simulink model "Hospital_Context"  (R2025b)
settings: Solver=VariableStepAuto  StartTime=0.0  StopTime=10.0  RelTol=1e-3
settings Model: Creator=jakeo  LastModifiedBy=jakeo

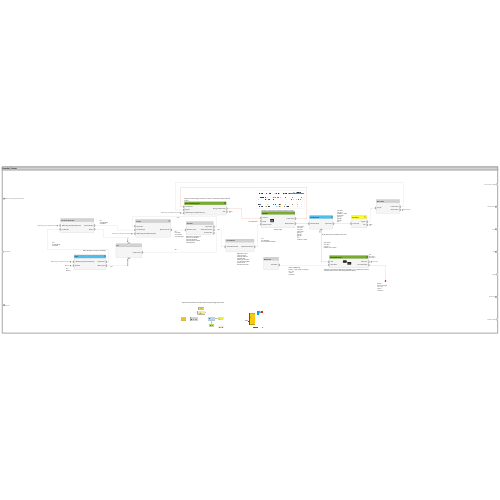
[thumbnail: Simulink's stored preview of the top-level diagram]
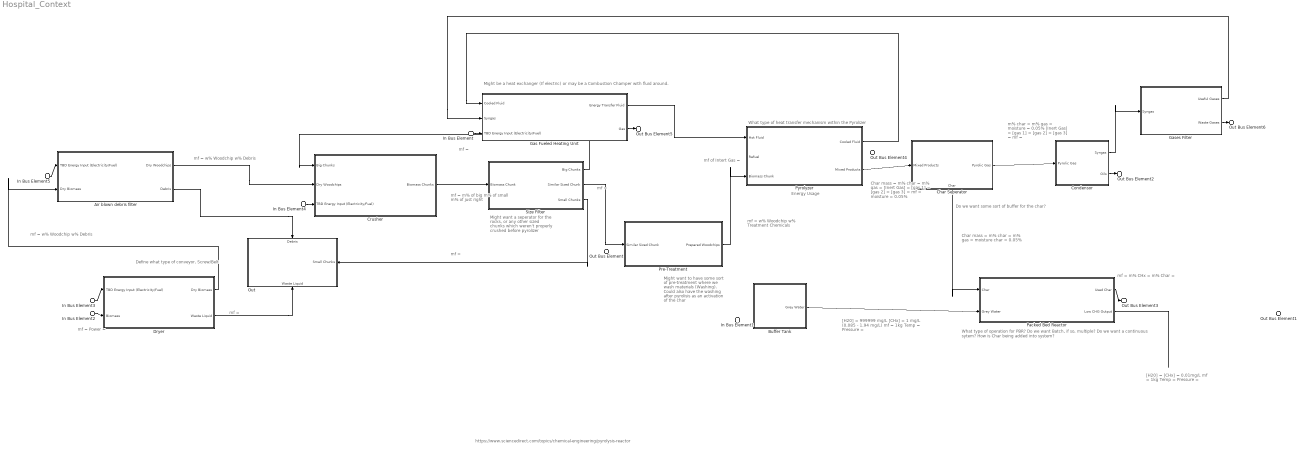
== system Hospital_Context ==
  note: mf =
      | m% CHx =
      | m% Char =
  note: Energy Usage
  note: mf of Intert Gas =
  note: m% char =
      | m% gas =
      | moisture = 0.05%
      | [Inert Gas] =
      | [gas 1] =
      | [gas 2] =
      | [gas 3] =
      | mf =
  note: Char mass =
      | m% char =
      | m% gas =
      | moisture char = 0.05%
  note: mf =
      | Power =
  note: Might want to have some sort of pre-treatment where we wash materials (Washing). Could also have the washing after pyrolisis as an activation of the char
  note: Do we want some sort of buffer for the char?
  note: What type of operation for PBR? Do we want Batch, if so, multiple? Do we want a continuous sytem? How is Char being added into system?
  note: Might want a seperator for the rocks, or any other sized chunks which weren't properly crushed before pyrolizer
  note: What type of heat transfer mechanism within the Pyrolizer
  note: Define what type of conveyor, Screw/Belt
  note: Might be a heat exchanger (If electric) or may be a Combustion Champer with fluid around.
  note: https://www.sciencedirect.com/topics/chemical-engineering/pyrolysis-reactor
  note: [H20] = 999999 mg/L
      | [CHx] = 1 mg/L  (0.085 - 1.94 mg/L)
      | mf = 1kg
      | Temp =
      | Pressure =
  note: [H20] =
      | [CHx] = 0.01mg/L
      | mf = 1kg
      | Temp =
      | Pressure =
  note: mf =
  note: mf =
      | w% Woodchip
      | w% Debris
  note: mf =
      | w% Woodchip
      | w% Debris
  note: Char mass =
      | m% char =
      | m% gas =
      | [Inert Gas] =
      | [gas 1] =
      | [gas 2] =
      | [gas 3] =
      | mf =
      | moisture = 0.05%
  note: mf =
      | m% of big
      | m% of small
      | m% of just right
  note: mf =
  note: mf =
      | w% Woodchip
      | w% Treatment Chemicals
  note: mf =
  note: mf =
  In Bus Element{,3..5} (4 alike) : Inport  PortName=TBD Energy Input (Electricity/Fuel)
  In Bus Element1 : Inport  Port=2  PortName=Grey Water 1
  In Bus Element2 : Inport  Port=3  PortName=Biomass
  Air blown debris filter : Subsystem
      settings: PortSchema="{\"entries\":[{\"content\":{\"headerSize\":26,\"margin\":15,\"minimumSpacing\":25,\"sides\":[{\"content\":{\"connectorIds\":[\"In2\",\"In1\"]},\"type\":\"ConnectorPlacement.EquallySpacedRectSide\",\"uuid\":\"cf9b5b84-c27e-443d-b9a2-3608ba31f5e4\"},{\"content\":{\"connectorIds\":[\"Out1\",\"Out2\"],\"side\":\"RIGHT\"},\"type\":\"ConnectorPlacement.EquallySpacedRectSide\",\"uuid\":\"efa89936-2b13-4422-9975-be719059dbdc\"},{\"content\":{\"side\":\"TOP\"},\"type\":\"ConnectorPlacement.EquallySpacedRectSide\",\"uuid\":\"249a79e9-4422-4697-8fba-0436c9decabf\"},{\"content\":{\"side\":\"BOTTOM\"},\"type\":\"ConnectorPlacement.EquallySpacedRectSide\",\"uuid\":\"86a2852a-f48b-482a-862b-0840c2ecc386\"}]},\"type\":\"ConnectorPlacement.EquallySpacedConnector\",\"uuid\":\"9d78504a-b513-4a9b-89b2-eac19dc7bc23\"}],\"packageUris\":[\"http://schema.mathworks.com/mf0/Connector/R2020b\"],\"version\":\"1.0\"}"
  Buffer Tank : Subsystem
      settings: PortSchema="{\"entries\":[{\"content\":{\"headerSize\":26,\"margin\":15,\"minimumSpacing\":25,\"sides\":[{\"content\":{},\"type\":\"ConnectorPlacement.EquallySpacedRectSide\",\"uuid\":\"cf9b5b84-c27e-443d-b9a2-3608ba31f5e4\"},{\"content\":{\"connectorIds\":[\"Out1\"],\"side\":\"RIGHT\"},\"type\":\"ConnectorPlacement.EquallySpacedRectSide\",\"uuid\":\"efa89936-2b13-4422-9975-be719059dbdc\"},{\"content\":{\"side\":\"TOP\"},\"type\":\"ConnectorPlacement.EquallySpacedRectSide\",\"uuid\":\"249a79e9-4422-4697-8fba-0436c9decabf\"}]},\"type\":\"ConnectorPlacement.EquallySpacedConnector\",\"uuid\":\"9d78504a-b513-4a9b-89b2-eac19dc7bc23\"}],\"packageUris\":[\"http://schema.mathworks.com/mf0/Connector/R2020b\"],\"version\":\"1.0\"}"
  Char Seperator : Subsystem
      settings: PortSchema="{\"entries\":[{\"content\":{\"headerSize\":26,\"margin\":15,\"minimumSpacing\":25,\"sides\":[{\"content\":{\"connectorIds\":[\"In1\"]},\"type\":\"ConnectorPlacement.EquallySpacedRectSide\",\"uuid\":\"fa1dbd3d-b57d-47b9-b4ef-0fe90e72294f\"},{\"content\":{\"connectorIds\":[\"Out1\"],\"side\":\"RIGHT\"},\"type\":\"ConnectorPlacement.EquallySpacedRectSide\",\"uuid\":\"948d51fa-2dfa-4f43-89d3-5e64c8759b0a\"},{\"content\":{\"side\":\"TOP\"},\"type\":\"ConnectorPlacement.EquallySpacedRectSide\",\"uuid\":\"ae7cb2a6-ad1d-4ea0-b46a-3d468529a90e\"},{\"content\":{\"connectorIds\":[\"Out2\"],\"side\":\"BOTTOM\"},\"type\":\"ConnectorPlacement.EquallySpacedRectSide\",\"uuid\":\"a440eaf4-fb0e-4071-9eb7-73669642cd6c\"}]},\"type\":\"ConnectorPlacement.EquallySpacedConnector\",\"uuid\":\"9e4666f3-ab23-41a5-b5e5-84e2e52e58ec\"}],\"packageUris\":[\"http://schema.mathworks.com/mf0/Connector/R2020b\"],\"version\":\"1.0\"}"
  Condensor : Subsystem
      settings: PortSchema="{\"entries\":[{\"content\":{\"headerSize\":26,\"margin\":15,\"minimumSpacing\":25,\"sides\":[{\"content\":{\"connectorIds\":[\"In1\"]},\"type\":\"ConnectorPlacement.EquallySpacedRectSide\",\"uuid\":\"fa1dbd3d-b57d-47b9-b4ef-0fe90e72294f\"},{\"content\":{\"connectorIds\":[\"Out1\",\"Out2\"],\"side\":\"RIGHT\"},\"type\":\"ConnectorPlacement.EquallySpacedRectSide\",\"uuid\":\"948d51fa-2dfa-4f43-89d3-5e64c8759b0a\"},{\"content\":{\"side\":\"TOP\"},\"type\":\"ConnectorPlacement.EquallySpacedRectSide\",\"uuid\":\"ae7cb2a6-ad1d-4ea0-b46a-3d468529a90e\"}]},\"type\":\"ConnectorPlacement.EquallySpacedConnector\",\"uuid\":\"9e4666f3-ab23-41a5-b5e5-84e2e52e58ec\"}],\"packageUris\":[\"http://schema.mathworks.com/mf0/Connector/R2020b\"],\"version\":\"1.0\"}"
  Crusher : Subsystem
      settings: PortSchema="{\"entries\":[{\"content\":{\"headerSize\":26,\"margin\":15,\"minimumSpacing\":25,\"sides\":[{\"content\":{\"connectorIds\":[\"In1\",\"In2\",\"In3\"]},\"type\":\"ConnectorPlacement.EquallySpacedRectSide\",\"uuid\":\"fa1dbd3d-b57d-47b9-b4ef-0fe90e72294f\"},{\"content\":{\"connectorIds\":[\"Out1\"],\"side\":\"RIGHT\"},\"type\":\"ConnectorPlacement.EquallySpacedRectSide\",\"uuid\":\"948d51fa-2dfa-4f43-89d3-5e64c8759b0a\"},{\"content\":{\"side\":\"TOP\"},\"type\":\"ConnectorPlacement.EquallySpacedRectSide\",\"uuid\":\"ae7cb2a6-ad1d-4ea0-b46a-3d468529a90e\"}]},\"type\":\"ConnectorPlacement.EquallySpacedConnector\",\"uuid\":\"9e4666f3-ab23-41a5-b5e5-84e2e52e58ec\"}],\"packageUris\":[\"http://schema.mathworks.com/mf0/Connector/R2020b\"],\"version\":\"1.0\"}"
  Dryer : Subsystem
      settings: PortSchema="{\"entries\":[{\"content\":{\"headerSize\":26,\"margin\":15,\"minimumSpacing\":25,\"sides\":[{\"content\":{\"connectorIds\":[\"In1\",\"In2\"]},\"type\":\"ConnectorPlacement.EquallySpacedRectSide\",\"uuid\":\"fa1dbd3d-b57d-47b9-b4ef-0fe90e72294f\"},{\"content\":{\"connectorIds\":[\"Out1\",\"Out2\"],\"side\":\"RIGHT\"},\"type\":\"ConnectorPlacement.EquallySpacedRectSide\",\"uuid\":\"948d51fa-2dfa-4f43-89d3-5e64c8759b0a\"},{\"content\":{\"side\":\"TOP\"},\"type\":\"ConnectorPlacement.EquallySpacedRectSide\",\"uuid\":\"ae7cb2a6-ad1d-4ea0-b46a-3d468529a90e\"}]},\"type\":\"ConnectorPlacement.EquallySpacedConnector\",\"uuid\":\"9e4666f3-ab23-41a5-b5e5-84e2e52e58ec\"}],\"packageUris\":[\"http://schema.mathworks.com/mf0/Connector/R2020b\"],\"version\":\"1.0\"}"
  Gas Fueled Heating Unit : Subsystem
      settings: PortSchema="{\"entries\":[{\"content\":{\"headerSize\":26,\"margin\":15,\"minimumSpacing\":25,\"sides\":[{\"content\":{\"connectorIds\":[\"In2\",\"In1\",\"In3\"]},\"type\":\"ConnectorPlacement.EquallySpacedRectSide\",\"uuid\":\"fa1dbd3d-b57d-47b9-b4ef-0fe90e72294f\"},{\"content\":{\"connectorIds\":[\"Out1\",\"Out2\"],\"side\":\"RIGHT\"},\"type\":\"ConnectorPlacement.EquallySpacedRectSide\",\"uuid\":\"948d51fa-2dfa-4f43-89d3-5e64c8759b0a\"},{\"content\":{\"side\":\"TOP\"},\"type\":\"ConnectorPlacement.EquallySpacedRectSide\",\"uuid\":\"ae7cb2a6-ad1d-4ea0-b46a-3d468529a90e\"}]},\"type\":\"ConnectorPlacement.EquallySpacedConnector\",\"uuid\":\"9e4666f3-ab23-41a5-b5e5-84e2e52e58ec\"}],\"packageUris\":[\"http://schema.mathworks.com/mf0/Connector/R2020b\"],\"version\":\"1.0\"}"
  Gases Filter : Subsystem
      settings: PortSchema="{\"entries\":[{\"content\":{\"headerSize\":26,\"margin\":15,\"minimumSpacing\":25,\"sides\":[{\"content\":{\"connectorIds\":[\"In1\"]},\"type\":\"ConnectorPlacement.EquallySpacedRectSide\",\"uuid\":\"cf9b5b84-c27e-443d-b9a2-3608ba31f5e4\"},{\"content\":{\"connectorIds\":[\"Out1\",\"Out2\"],\"side\":\"RIGHT\"},\"type\":\"ConnectorPlacement.EquallySpacedRectSide\",\"uuid\":\"efa89936-2b13-4422-9975-be719059dbdc\"},{\"content\":{\"side\":\"TOP\"},\"type\":\"ConnectorPlacement.EquallySpacedRectSide\",\"uuid\":\"249a79e9-4422-4697-8fba-0436c9decabf\"}]},\"type\":\"ConnectorPlacement.EquallySpacedConnector\",\"uuid\":\"9d78504a-b513-4a9b-89b2-eac19dc7bc23\"}],\"packageUris\":[\"http://schema.mathworks.com/mf0/Connector/R2020b\"],\"version\":\"1.0\"}"
  Out : Subsystem
      settings: PortSchema="{\"entries\":[{\"content\":{\"headerSize\":26,\"margin\":15,\"minimumSpacing\":25,\"sides\":[{\"content\":{},\"type\":\"ConnectorPlacement.EquallySpacedRectSide\",\"uuid\":\"cf9b5b84-c27e-443d-b9a2-3608ba31f5e4\"},{\"content\":{\"connectorIds\":[\"In2\"],\"side\":\"RIGHT\"},\"type\":\"ConnectorPlacement.EquallySpacedRectSide\",\"uuid\":\"efa89936-2b13-4422-9975-be719059dbdc\"},{\"content\":{\"connectorIds\":[\"In3\"],\"side\":\"TOP\"},\"type\":\"ConnectorPlacement.EquallySpacedRectSide\",\"uuid\":\"249a79e9-4422-4697-8fba-0436c9decabf\"},{\"content\":{\"connectorIds\":[\"In1\"],\"side\":\"BOTTOM\"},\"type\":\"ConnectorPlacement.EquallySpacedRectSide\",\"uuid\":\"a2f86060-a3f0-4067-b3c8-949b6bb1e736\"}]},\"type\":\"ConnectorPlacement.EquallySpacedConnector\",\"uuid\":\"9d78504a-b513-4a9b-89b2-eac19dc7bc23\"}],\"packageUris\":[\"http://schema.mathworks.com/mf0/Connector/R2020b\"],\"version\":\"1.0\"}"
  Packed Bed Reactor : Subsystem
      settings: PortSchema="{\"entries\":[{\"content\":{\"headerSize\":26,\"margin\":15,\"minimumSpacing\":25,\"sides\":[{\"content\":{\"connectorIds\":[\"In1\",\"In2\"]},\"type\":\"ConnectorPlacement.EquallySpacedRectSide\",\"uuid\":\"fa1dbd3d-b57d-47b9-b4ef-0fe90e72294f\"},{\"content\":{\"connectorIds\":[\"Out2\",\"Out1\"],\"side\":\"RIGHT\"},\"type\":\"ConnectorPlacement.EquallySpacedRectSide\",\"uuid\":\"948d51fa-2dfa-4f43-89d3-5e64c8759b0a\"},{\"content\":{\"side\":\"TOP\"},\"type\":\"ConnectorPlacement.EquallySpacedRectSide\",\"uuid\":\"ae7cb2a6-ad1d-4ea0-b46a-3d468529a90e\"},{\"content\":{\"side\":\"BOTTOM\"},\"type\":\"ConnectorPlacement.EquallySpacedRectSide\",\"uuid\":\"dc29dfe4-3980-46f5-bd0d-b60b93a30b71\"}]},\"type\":\"ConnectorPlacement.EquallySpacedConnector\",\"uuid\":\"9e4666f3-ab23-41a5-b5e5-84e2e52e58ec\"}],\"packageUris\":[\"http://schema.mathworks.com/mf0/Connector/R2020b\"],\"version\":\"1.0\"}"
  Pre-Treatment : Subsystem
      settings: PortSchema="{\"entries\":[{\"content\":{\"headerSize\":26,\"margin\":15,\"minimumSpacing\":25,\"sides\":[{\"content\":{\"connectorIds\":[\"In1\"]},\"type\":\"ConnectorPlacement.EquallySpacedRectSide\",\"uuid\":\"cf9b5b84-c27e-443d-b9a2-3608ba31f5e4\"},{\"content\":{\"connectorIds\":[\"Out1\"],\"side\":\"RIGHT\"},\"type\":\"ConnectorPlacement.EquallySpacedRectSide\",\"uuid\":\"efa89936-2b13-4422-9975-be719059dbdc\"},{\"content\":{\"side\":\"TOP\"},\"type\":\"ConnectorPlacement.EquallySpacedRectSide\",\"uuid\":\"249a79e9-4422-4697-8fba-0436c9decabf\"}]},\"type\":\"ConnectorPlacement.EquallySpacedConnector\",\"uuid\":\"9d78504a-b513-4a9b-89b2-eac19dc7bc23\"}],\"packageUris\":[\"http://schema.mathworks.com/mf0/Connector/R2020b\"],\"version\":\"1.0\"}"
  Pyrolyzer : Subsystem
      settings: PortSchema="{\"entries\":[{\"content\":{\"headerSize\":26,\"margin\":15,\"minimumSpacing\":25,\"sides\":[{\"content\":{\"connectorIds\":[\"In3\",\"In2\",\"In1\"]},\"type\":\"ConnectorPlacement.EquallySpacedRectSide\",\"uuid\":\"fa1dbd3d-b57d-47b9-b4ef-0fe90e72294f\"},{\"content\":{\"connectorIds\":[\"Out1\",\"Out2\"],\"side\":\"RIGHT\"},\"type\":\"ConnectorPlacement.EquallySpacedRectSide\",\"uuid\":\"948d51fa-2dfa-4f43-89d3-5e64c8759b0a\"},{\"content\":{\"side\":\"TOP\"},\"type\":\"ConnectorPlacement.EquallySpacedRectSide\",\"uuid\":\"ae7cb2a6-ad1d-4ea0-b46a-3d468529a90e\"},{\"content\":{\"side\":\"BOTTOM\"},\"type\":\"ConnectorPlacement.EquallySpacedRectSide\",\"uuid\":\"c41ca62f-2536-4c7c-93b5-233085d0098c\"}]},\"type\":\"ConnectorPlacement.EquallySpacedConnector\",\"uuid\":\"9e4666f3-ab23-41a5-b5e5-84e2e52e58ec\"}],\"packageUris\":[\"http://schema.mathworks.com/mf0/Connector/R2020b\"],\"version\":\"1.0\"}"
  Size Filter : Subsystem
      settings: PortSchema="{\"entries\":[{\"content\":{\"headerSize\":26,\"margin\":15,\"minimumSpacing\":25,\"sides\":[{\"content\":{\"connectorIds\":[\"In1\"]},\"type\":\"ConnectorPlacement.EquallySpacedRectSide\",\"uuid\":\"cf9b5b84-c27e-443d-b9a2-3608ba31f5e4\"},{\"content\":{\"connectorIds\":[\"Out1\",\"Out2\",\"Out3\"],\"side\":\"RIGHT\"},\"type\":\"ConnectorPlacement.EquallySpacedRectSide\",\"uuid\":\"efa89936-2b13-4422-9975-be719059dbdc\"},{\"content\":{\"side\":\"TOP\"},\"type\":\"ConnectorPlacement.EquallySpacedRectSide\",\"uuid\":\"249a79e9-4422-4697-8fba-0436c9decabf\"}]},\"type\":\"ConnectorPlacement.EquallySpacedConnector\",\"uuid\":\"9d78504a-b513-4a9b-89b2-eac19dc7bc23\"}],\"packageUris\":[\"http://schema.mathworks.com/mf0/Connector/R2020b\"],\"version\":\"1.0\"}"
  Out Bus Element1 : Outport  PortName=Low CHG Grey Water
  Out Bus Element6 : Outport  Port=2  PortName=Waste Gases
  Out Bus Element5 : Outport  Port=3  PortName=Gas
  Out Bus Element2 : Outport  Port=4  PortName=Oils
  Out Bus Element : Outport  Port=5  PortName=Sludge
  Out Bus Element3 : Outport  Port=6  PortName=Used Char
  Out Bus Element4 : Outport  Port=7  PortName=Biomass Waste
  wires:
  Pyrolyzer/2(Mixed Products) -> Char Seperator/1(Mixed Products)
  Packed Bed Reactor/2(Used Char) -> Out Bus Element3/1
  Packed Bed Reactor/1(Low CHG Output) -> ?
  Buffer Tank/1(Grey Water) -> Packed Bed Reactor/2(Grey Water)
  In Bus Element2/1 -> Dryer/2(Biomass)
  Dryer/1(Dry Biomass) -> Air blown debris filter/1(Dry Biomass)
  Crusher/1(Biomass Chunks) -> Size Filter/1(Biomass Chunk)
  In Bus Element/1 -> Gas Fueled Heating Unit/3(TBD Energy Input (Electricity/Fuel))
  Gas Fueled Heating Unit/1(Energy Transfer Fluid) -> Pyrolyzer/3(Hot Fluid)
  Char Seperator/2(Char) -> Packed Bed Reactor/1(Char)
  Dryer/2(Waste Liquid) -> Out/1(Waste Liquid)
  Char Seperator/1(Pyrolic Gas) -> Condensor/1(Pyrolic Gas)
  Condensor/2(Oils) -> Out Bus Element2/1
  In Bus Element3/1 -> Dryer/1(TBD Energy Input (Electricity/Fuel))
  In Bus Element4/1 -> Crusher/3(TBD Energy Input (Electricity/Fuel))
  In Bus Element5/1 -> Air blown debris filter/2(TBD Energy Input (Electricity/Fuel))
  Air blown debris filter/1(Dry Woodchips) -> Crusher/2(Dry Woodchips)
  Air blown debris filter/2(Debris) -> Out/3(Debris)
  Pyrolyzer/1(Cooled Fluid) -> Gas Fueled Heating Unit/2(Cooled Fluid)
  Size Filter/2(Similar Sized Chunk) -> Pre-Treatment/1(Similar Sized Chunk)
  Pre-Treatment/1(Prepared Woodchips) -> Pyrolyzer/1(Biomass Chunk)
  Size Filter/1(Big Chunks) -> Crusher/1(Big Chunks)
  Size Filter/3(Small Chunks) -> Out/2(Small Chunks)
  Gas Fueled Heating Unit/2(Gas) -> Out Bus Element5/1
  Condensor/1(Syngas) -> Gases Filter/1(Syngas)
  Gases Filter/2(Waste Gases) -> Out Bus Element6/1
  Gases Filter/1(Useful Gases) -> Gas Fueled Heating Unit/1(Syngas)

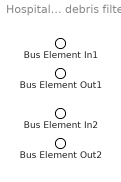
== system Hospital_Context/Air blown debris filter ==
  Bus Element In1 : Inport  PortName=Dry Biomass
  Bus Element In2 : Inport  Port=2  PortName=TBD Energy Input (Electricity/Fuel)
  Bus Element Out1 : Outport  PortName=Dry Woodchips
  Bus Element Out2 : Outport  Port=2  PortName=Debris

== system Hospital_Context/Buffer Tank ==
  Bus Element Out1 : Outport  PortName=Grey Water

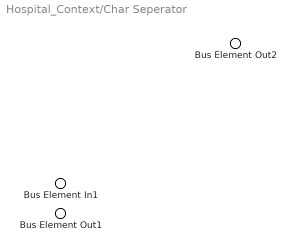
== system Hospital_Context/Char Seperator ==
  Bus Element In1 : Inport  PortName=Mixed Products
  Bus Element Out2 : Outport  PortName=Pyrolic Gas
  Bus Element Out1 : Outport  Port=2  PortName=Char

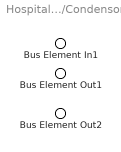
== system Hospital_Context/Condensor ==
  Bus Element In1 : Inport  PortName=Pyrolic Gas
  Bus Element Out1 : Outport  PortName=Syngas
  Bus Element Out2 : Outport  Port=2  PortName=Oils

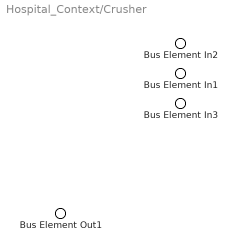
== system Hospital_Context/Crusher ==
  Bus Element In3 : Inport  PortName=Big Chunks
  Bus Element In1 : Inport  Port=2  PortName=Dry Woodchips
  Bus Element In2 : Inport  Port=3  PortName=TBD Energy Input (Electricity/Fuel)
  Bus Element Out1 : Outport  PortName=Biomass Chunks

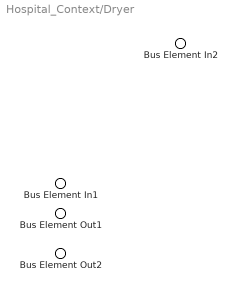
== system Hospital_Context/Dryer ==
  Bus Element In2 : Inport  PortName=TBD Energy Input (Electricity/Fuel)
  Bus Element In1 : Inport  Port=2  PortName=Biomass
  Bus Element Out1 : Outport  PortName=Dry Biomass
  Bus Element Out2 : Outport  Port=2  PortName=Waste Liquid

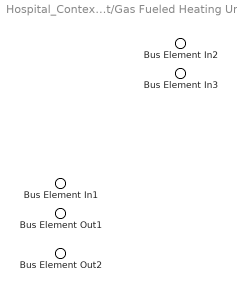
== system Hospital_Context/Gas Fueled Heating Unit ==
  Bus Element In3 : Inport  PortName=Syngas
  Bus Element In2 : Inport  Port=2  PortName=Cooled Fluid
  Bus Element In1 : Inport  Port=3  PortName=TBD Energy Input (Electricity/Fuel)
  Bus Element Out1 : Outport  PortName=Energy Transfer Fluid
  Bus Element Out2 : Outport  Port=2  PortName=Gas

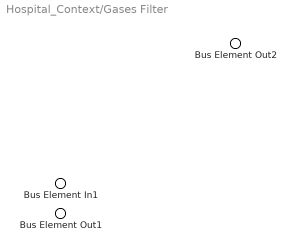
== system Hospital_Context/Gases Filter ==
  Bus Element In1 : Inport  PortName=Syngas
  Bus Element Out2 : Outport  PortName=Useful Gases
  Bus Element Out1 : Outport  Port=2  PortName=Waste Gases

== system Hospital_Context/Out ==
  Bus Element In3 : Inport  PortName=Waste Liquid
  Bus Element In2 : Inport  Port=2  PortName=Small Chunks
  Bus Element In1 : Inport  Port=3  PortName=Debris

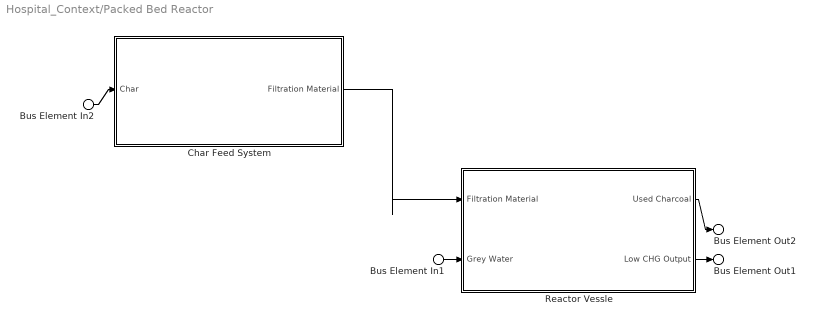
== system Hospital_Context/Packed Bed Reactor ==
  Bus Element In2 : Inport  PortName=Char
  Bus Element In1 : Inport  Port=2  PortName=Grey Water
  Char Feed System : Subsystem
      settings: PortSchema="{\"entries\":[{\"content\":{\"headerSize\":26,\"margin\":15,\"minimumSpacing\":25,\"sides\":[{\"content\":{\"connectorIds\":[\"In1\"]},\"type\":\"ConnectorPlacement.EquallySpacedRectSide\",\"uuid\":\"fa1dbd3d-b57d-47b9-b4ef-0fe90e72294f\"},{\"content\":{\"connectorIds\":[\"Out1\"],\"side\":\"RIGHT\"},\"type\":\"ConnectorPlacement.EquallySpacedRectSide\",\"uuid\":\"948d51fa-2dfa-4f43-89d3-5e64c8759b0a\"},{\"content\":{\"side\":\"TOP\"},\"type\":\"ConnectorPlacement.EquallySpacedRectSide\",\"uuid\":\"ae7cb2a6-ad1d-4ea0-b46a-3d468529a90e\"}]},\"type\":\"ConnectorPlacement.EquallySpacedConnector\",\"uuid\":\"9e4666f3-ab23-41a5-b5e5-84e2e52e58ec\"}],\"packageUris\":[\"http://schema.mathworks.com/mf0/Connector/R2020b\"],\"version\":\"1.0\"}"
  Reactor Vessle : Subsystem
      settings: PortSchema="{\"entries\":[{\"content\":{\"headerSize\":26,\"margin\":15,\"minimumSpacing\":25,\"sides\":[{\"content\":{\"connectorIds\":[\"In1\",\"In2\"]},\"type\":\"ConnectorPlacement.EquallySpacedRectSide\",\"uuid\":\"fa1dbd3d-b57d-47b9-b4ef-0fe90e72294f\"},{\"content\":{\"connectorIds\":[\"Out1\",\"Out2\"],\"side\":\"RIGHT\"},\"type\":\"ConnectorPlacement.EquallySpacedRectSide\",\"uuid\":\"948d51fa-2dfa-4f43-89d3-5e64c8759b0a\"},{\"content\":{\"side\":\"TOP\"},\"type\":\"ConnectorPlacement.EquallySpacedRectSide\",\"uuid\":\"ae7cb2a6-ad1d-4ea0-b46a-3d468529a90e\"}]},\"type\":\"ConnectorPlacement.EquallySpacedConnector\",\"uuid\":\"9e4666f3-ab23-41a5-b5e5-84e2e52e58ec\"}],\"packageUris\":[\"http://schema.mathworks.com/mf0/Connector/R2020b\"],\"version\":\"1.0\"}"
  Bus Element Out1 : Outport  PortName=Low CHG Output
  Bus Element Out2 : Outport  Port=2  PortName=Used Char
  wires:
  Bus Element In1/1 -> Reactor Vessle/2(Grey Water)
  Char Feed System/1(Filtration Material) -> Reactor Vessle/1(Filtration Material)
  Reactor Vessle/1(Used Charcoal) -> Bus Element Out2/1
  Reactor Vessle/2(Low CHG Output) -> Bus Element Out1/1
  Bus Element In2/1 -> Char Feed System/1(Char)

== system Hospital_Context/Pre-Treatment ==
  Bus Element In1 : Inport  PortName=Similar Sized Chunk
  Bus Element Out1 : Outport  PortName=Prepared Woodchips

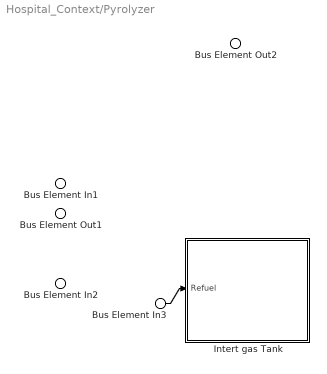
== system Hospital_Context/Pyrolyzer ==
  Bus Element In1 : Inport  PortName=Biomass Chunk
  Bus Element In3 : Inport  Port=2  PortName=Refuel
  Bus Element In2 : Inport  Port=3  PortName=Hot Fluid
  Intert gas Tank : Subsystem
      settings: PortSchema="{\"entries\":[{\"content\":{\"headerSize\":26,\"margin\":15,\"minimumSpacing\":25,\"sides\":[{\"content\":{\"connectorIds\":[\"In1\"]},\"type\":\"ConnectorPlacement.EquallySpacedRectSide\",\"uuid\":\"cf9b5b84-c27e-443d-b9a2-3608ba31f5e4\"},{\"content\":{\"side\":\"RIGHT\"},\"type\":\"ConnectorPlacement.EquallySpacedRectSide\",\"uuid\":\"efa89936-2b13-4422-9975-be719059dbdc\"},{\"content\":{\"side\":\"TOP\"},\"type\":\"ConnectorPlacement.EquallySpacedRectSide\",\"uuid\":\"249a79e9-4422-4697-8fba-0436c9decabf\"}]},\"type\":\"ConnectorPlacement.EquallySpacedConnector\",\"uuid\":\"9d78504a-b513-4a9b-89b2-eac19dc7bc23\"}],\"packageUris\":[\"http://schema.mathworks.com/mf0/Connector/R2020b\"],\"version\":\"1.0\"}"
  Bus Element Out2 : Outport  PortName=Cooled Fluid
  Bus Element Out1 : Outport  Port=2  PortName=Mixed Products
  wires:
  Bus Element In3/1 -> Intert gas Tank/1(Refuel)

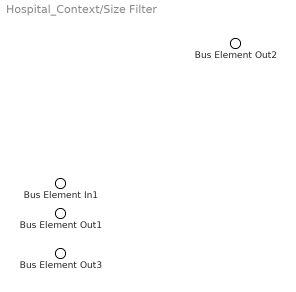
== system Hospital_Context/Size Filter ==
  Bus Element In1 : Inport  PortName=Biomass Chunk
  Bus Element Out2 : Outport  PortName=Big Chunks
  Bus Element Out1 : Outport  Port=2  PortName=Similar Sized Chunk
  Bus Element Out3 : Outport  Port=3  PortName=Small Chunks

== system Hospital_Context/Packed Bed Reactor/Char Feed System ==
  Bus Element In1 : Inport  PortName=Char
  Bus Element Out1 : Outport  PortName=Filtration Material

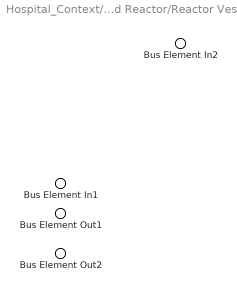
== system Hospital_Context/Packed Bed Reactor/Reactor Vessle ==
  Bus Element In2 : Inport  PortName=Filtration Material
  Bus Element In1 : Inport  Port=2  PortName=Grey Water
  Bus Element Out1 : Outport  PortName=Used Charcoal
  Bus Element Out2 : Outport  Port=2  PortName=Low CHG Output

== system Hospital_Context/Pyrolyzer/Intert gas Tank ==
  Bus Element In1 : Inport  PortName=Refuel
